simulink model "template_Final_Project_MPC5643L"  (Simulink 7.8)
settings: Solver=FixedStepDiscrete  StartTime=0.0  StopTime=10.0  RelTol=1e-3
InitFcn:
  | parameters
values from neighbouring files (symbols this model uses):
  Ak = 100    [parameters.m]
  b = 100    [parameters.m]
  dT = 0.01    [parameters.m]
  H = 10    [parameters.m]
  Kd_PD = 0.04    [parameters.m]
  Kd_PID = 40    [parameters.m]
  Ki_PID = 0    [parameters.m]
  Kp_PD = 0.4    [parameters.m]
  Kp_PID = 500    [parameters.m]
  L1 = 1.6    [parameters.m]
  L2 = 0.8    [parameters.m]
  m = 2000    [parameters.m]
  V_Ki = 50    [parameters.m]
  V_Kp = 5000    [parameters.m]
undefined symbols (not defined in the file or in its folder): A10, A13, A14, A7, A8, AN0, B, B13, B4, B6, B7, B8, C5, C6, D, D11, D4, DiscIntNeverNeededParam, F15, F3, F4, G4, H4, L3, M14, M3, N15, N3, P3, PA10, PA11, PA12, PA13, PA14, PA5, PA6, PA7, PA8, PA9, PB13, PB7, PC11, PC12, PC13, PC14, PC15, PC6, PD0, PD1, PD10, PD11, PD2, PD3, PD4, PD5, PD6, PD7, PD8, PD9, R10 ... (+4)
libraries: Conv_Lib x54, rappid_564xl_ec_toolbox x50, simulink x19, Veh_Sim x9, U_of_M_5643_blockset x1
(part 2 of 2)

== system template_Final_Project_MPC5643L/High-Level Design/Inputs/Other Cars/Car5 ==
  Bytes to Single{,1..3} (4 alike) : Conv_Lib/Bytes to Single
  CAN_Receive_data : rappid_564xl_ec_toolbox/MPC564xL/Communication Blocks/CAN_Receive_data  can_unit=A  can_unit_v2=0  can_buffer=10  can_id=65
  CAN_Receive_data1 : rappid_564xl_ec_toolbox/MPC564xL/Communication Blocks/CAN_Receive_data  can_unit=A  can_unit_v2=0  can_buffer=11  can_id=66
  Demux : Demux  Outputs=2
  Demux1 : Demux  Outputs=2
  Mux : Mux
  Terminator{,1..5} (6 alike) : Terminator
  s,n,psi,us : Outport
  wires:
  Bytes to Single1/1 -> Mux/2
  Bytes to Single3/1 -> Mux/3
  Demux/1 -> Bytes to Single/1
  Demux/2 -> Bytes to Single1/1
  Demux1/1 -> Bytes to Single2/1
  Demux1/2 -> Bytes to Single3/1
  Bytes to Single/1 -> Mux/1
  Bytes to Single2/1 -> Mux/4
  Mux/1 -> s,n,psi,us/1
  CAN_Receive_data/1 -> Terminator/1
  CAN_Receive_data/2 -> Terminator1/1
  CAN_Receive_data/3 -> Demux/1
  CAN_Receive_data/4 -> Terminator2/1
  CAN_Receive_data1/1 -> Terminator3/1
  CAN_Receive_data1/2 -> Terminator4/1
  CAN_Receive_data1/3 -> Demux1/1
  CAN_Receive_data1/4 -> Terminator5/1

== system template_Final_Project_MPC5643L/High-Level Design/Inputs/Other Cars/Car6 ==
  Bytes to Single{,1..3} (4 alike) : Conv_Lib/Bytes to Single
  CAN_Receive_data : rappid_564xl_ec_toolbox/MPC564xL/Communication Blocks/CAN_Receive_data  can_unit=A  can_unit_v2=0  can_buffer=12  can_id=55
  CAN_Receive_data1 : rappid_564xl_ec_toolbox/MPC564xL/Communication Blocks/CAN_Receive_data  can_unit=A  can_unit_v2=0  can_buffer=13  can_id=56
  Demux : Demux  Outputs=2
  Demux1 : Demux  Outputs=2
  Mux : Mux
  Terminator{,1..5} (6 alike) : Terminator
  s,n,psi,us : Outport
  wires:
  CAN_Receive_data1/4 -> Terminator5/1
  CAN_Receive_data1/3 -> Demux1/1
  CAN_Receive_data1/2 -> Terminator4/1
  CAN_Receive_data1/1 -> Terminator3/1
  CAN_Receive_data/4 -> Terminator2/1
  CAN_Receive_data/3 -> Demux/1
  CAN_Receive_data/2 -> Terminator1/1
  CAN_Receive_data/1 -> Terminator/1
  Mux/1 -> s,n,psi,us/1
  Bytes to Single2/1 -> Mux/4
  Bytes to Single/1 -> Mux/1
  Demux1/2 -> Bytes to Single3/1
  Demux1/1 -> Bytes to Single2/1
  Demux/2 -> Bytes to Single1/1
  Demux/1 -> Bytes to Single/1
  Bytes to Single3/1 -> Mux/3
  Bytes to Single1/1 -> Mux/2

== system template_Final_Project_MPC5643L/High-Level Design/Inputs/Other Cars/GSI Car ==
  Bytes to Single{,1..3} (4 alike) : Conv_Lib/Bytes to Single
  CAN_Receive_data : rappid_564xl_ec_toolbox/MPC564xL/Communication Blocks/CAN_Receive_data  can_unit=A  can_unit_v2=0  can_buffer=0  can_id=0
  CAN_Receive_data1 : rappid_564xl_ec_toolbox/MPC564xL/Communication Blocks/CAN_Receive_data  can_unit=A  can_unit_v2=0  can_buffer=1  can_id=0
  Demux : Demux  Outputs=2
  Demux1 : Demux  Outputs=2
  Mux : Mux
  Terminator{,1..5} (6 alike) : Terminator
  s,n,psi,us : Outport
  wires:
  Bytes to Single1/1 -> Mux/2
  Bytes to Single3/1 -> Mux/3
  Demux/1 -> Bytes to Single/1
  Demux/2 -> Bytes to Single1/1
  Demux1/1 -> Bytes to Single2/1
  Demux1/2 -> Bytes to Single3/1
  Bytes to Single/1 -> Mux/1
  Bytes to Single2/1 -> Mux/4
  Mux/1 -> s,n,psi,us/1
  CAN_Receive_data/1 -> Terminator/1
  CAN_Receive_data/2 -> Terminator1/1
  CAN_Receive_data/3 -> Demux/1
  CAN_Receive_data/4 -> Terminator2/1
  CAN_Receive_data1/1 -> Terminator3/1
  CAN_Receive_data1/2 -> Terminator4/1
  CAN_Receive_data1/3 -> Demux1/1
  CAN_Receive_data1/4 -> Terminator5/1

== system template_Final_Project_MPC5643L/High-Level Design/Inputs/Other Cars/Zeros (20) ==
  Constant : Constant  Value=0  OutDataTypeStr=single
  Mux : Mux  Inputs=20
  Zeros : Outport
  wires:
  Constant/1 -> Mux/1, Mux/2, Mux/3, Mux/4, Mux/5, Mux/6, Mux/7, Mux/8, Mux/9, Mux/10, Mux/11, Mux/12, Mux/13, Mux/14, Mux/15, Mux/16, Mux/18, Mux/19, Mux/20, Mux/17
  Mux/1 -> Zeros/1

== system template_Final_Project_MPC5643L/High-Level Design/Outputs/Extract x,y,psi (Cars 1 - 6)/Extract x,y,psi ==
  s,n,psi,us : Inport
  Demux : Demux
  Mux : Mux  Inputs=3
  Terminator : Terminator
  s,n to x,y : Veh_Sim/s,n to x,y  SystemSampleTime=-1
  x,y,psi : Outport
  wires:
  Demux/1 -> s,n to x,y/1
  Demux/2 -> s,n to x,y/2
  s,n,psi,us/1 -> Demux/1
  s,n to x,y/1 -> Mux/1
  s,n to x,y/2 -> Mux/2
  Demux/3 -> Mux/3
  Mux/1 -> x,y,psi/1
  Demux/4 -> Terminator/1

== system template_Final_Project_MPC5643L/High-Level Design/Outputs/Extract x,y,psi (Cars 1 - 6)/Extract x,y,psi1 ==
  s,n,psi,us : Inport
  Demux : Demux
  Mux : Mux  Inputs=3
  Terminator : Terminator
  s,n to x,y : Veh_Sim/s,n to x,y  SystemSampleTime=-1
  x,y,psi : Outport
  wires:
  Demux/1 -> s,n to x,y/1
  Demux/2 -> s,n to x,y/2
  s,n,psi,us/1 -> Demux/1
  s,n to x,y/1 -> Mux/1
  s,n to x,y/2 -> Mux/2
  Demux/3 -> Mux/3
  Mux/1 -> x,y,psi/1
  Demux/4 -> Terminator/1

== system template_Final_Project_MPC5643L/High-Level Design/Outputs/Extract x,y,psi (Cars 1 - 6)/Extract x,y,psi2 ==
  s,n,psi,us : Inport
  Demux : Demux
  Mux : Mux  Inputs=3
  Terminator : Terminator
  s,n to x,y : Veh_Sim/s,n to x,y  SystemSampleTime=-1
  x,y,psi : Outport
  wires:
  Demux/1 -> s,n to x,y/1
  Demux/2 -> s,n to x,y/2
  s,n,psi,us/1 -> Demux/1
  s,n to x,y/1 -> Mux/1
  s,n to x,y/2 -> Mux/2
  Demux/3 -> Mux/3
  Mux/1 -> x,y,psi/1
  Demux/4 -> Terminator/1

== system template_Final_Project_MPC5643L/High-Level Design/Outputs/Extract x,y,psi (Cars 1 - 6)/Extract x,y,psi3 ==
  s,n,psi,us : Inport
  Demux : Demux
  Mux : Mux  Inputs=3
  Terminator : Terminator
  s,n to x,y : Veh_Sim/s,n to x,y  SystemSampleTime=-1
  x,y,psi : Outport
  wires:
  Demux/1 -> s,n to x,y/1
  Demux/2 -> s,n to x,y/2
  s,n,psi,us/1 -> Demux/1
  s,n to x,y/1 -> Mux/1
  s,n to x,y/2 -> Mux/2
  Demux/3 -> Mux/3
  Mux/1 -> x,y,psi/1
  Demux/4 -> Terminator/1

== system template_Final_Project_MPC5643L/High-Level Design/Outputs/Extract x,y,psi (Cars 1 - 6)/Extract x,y,psi4 ==
  s,n,psi,us : Inport
  Demux : Demux
  Mux : Mux  Inputs=3
  Terminator : Terminator
  s,n to x,y : Veh_Sim/s,n to x,y  SystemSampleTime=-1
  x,y,psi : Outport
  wires:
  Demux/1 -> s,n to x,y/1
  Demux/2 -> s,n to x,y/2
  s,n,psi,us/1 -> Demux/1
  s,n to x,y/1 -> Mux/1
  s,n to x,y/2 -> Mux/2
  Demux/3 -> Mux/3
  Mux/1 -> x,y,psi/1
  Demux/4 -> Terminator/1

== system template_Final_Project_MPC5643L/High-Level Design/Outputs/Extract x,y,psi (Cars 1 - 6)/Extract x,y,psi5 ==
  s,n,psi,us : Inport
  Demux : Demux
  Mux : Mux  Inputs=3
  Terminator : Terminator
  s,n to x,y : Veh_Sim/s,n to x,y  SystemSampleTime=-1
  x,y,psi : Outport
  wires:
  Demux/1 -> s,n to x,y/1
  Demux/2 -> s,n to x,y/2
  s,n,psi,us/1 -> Demux/1
  s,n to x,y/1 -> Mux/1
  s,n to x,y/2 -> Mux/2
  Demux/3 -> Mux/3
  Mux/1 -> x,y,psi/1
  Demux/4 -> Terminator/1

== system template_Final_Project_MPC5643L/High-Level Design/ACC/Speed Ctrl/PI/My Discrete Integrator ==
  X_dot : Inport
  Gain : Gain  Gain=dT  SaturateOnIntegerOverflow=on  OutDataTypeStr=Inherit: Same as input  ParamDataTypeStr=Inherit: Same as input
  Sum : Sum  Inputs=|++  SaturateOnIntegerOverflow=on  InputSameDT=on  OutDataTypeStr=Inherit: Same as first input
  Unit Delay : UnitDelay  SampleTime=-1
  X : Outport
  wires:
  Unit Delay/1 -> X/1, Sum/2
  Sum/1 -> Unit Delay/1
  X_dot/1 -> Gain/1
  Gain/1 -> Sum/1

== stateflow chart High-Level Design/ACC/ACC State Logic/Chart ==
  state PosCTRL
    during:
    speed_en=0;
    pos_en = 1;
    man_en=0;
    state=4;
  state SpeedCTRL
    during:
    speed_en=1;
    pos_en=0;
    man_en=0;
    state=2;
  state ManCTRL
    during:
    speed_en =0;
    pos_en=0;
    man_en=1;
    state =1;
  PosCTRL -> SpeedCTRL [order 1] : [((usi>us) || (si-s>H))]
  SpeedCTRL -> PosCTRL [order 1] : [((usi<=us) && (si-s<=H))]
  SpeedCTRL -> ManCTRL [order 2] : [enable]
  ManCTRL -> SpeedCTRL : [!enable]
  PosCTRL -> ManCTRL [order 2] : [enable]
  (default) -> ManCTRL
  data: enable input boolean; usi input double; si input double; us input double; s input double; H input double; speed_en output boolean; pos_en output boolean; man_en output boolean; state output single
